simulink model "cPegasusAutopilot"  (R2020a)
settings: Solver=ode4  StartTime=0.0  StopTime=inf  FixedStep=0.01  RelTol=1e-3  EnableMultiTasking=on
undefined symbols (not defined in the file or in its folder): f, Ue
libraries: xpcutilitieslib x4, instrumentlib x2, simulink x1
settings Model: PauseTimes=88  Creator=Marcelo Henrique  LastModifiedBy=adalb
settings DataIOCC: LimitDataPoints=on  SaveFormat=Array  ReturnWorkspaceOutputs=off
settings OptimizationCC: LifeSpan=inf
settings DebuggingCC: AlgebraicLoopMsg=none  UnderspecifiedInitializationDetection=Classic  MergeDetectMultiDrivingBlocksExec=none  StateNameClashWarn=warning  SFUnexpectedBacktrackingDiag=warning  SFNoUnconditionalDefaultTransitionDiag=warning  ArithmeticOperatorsInVariantConditions=warning
settings HardwareCC: ProdBitPerPointer=32  ProdBitPerSizeT=32  ProdBitPerPtrDiffT=32  ProdLargestAtomicFloat=None  ProdIntDivRoundTo=Undefined  ProdEndianess=Unspecified  ProdWordSize=32  ProdHWDeviceType=32-bit Generic
settings ModelReferenceCC: PropagateSignalLabelsOutOfModel=off
settings SFSimCC: SimUseLocalCustomCode=off  CustomCodeUndefinedFunction=UseInterfaceOnly
settings RTWCC: RTWUseLocalCustomCode=off
settings CodeAppCC: StateflowObjectComments=on
settings GRTTargetCC: TargetLangStandard=C89/C90 (ANSI)
settings ConfigComp: CovMetricSettings=dw  CovHtmlReporting=on  CovSaveCumulativeToWorkspaceVar=on  CovSaveSingleToWorkspaceVar=on  CovExternalEMLEnable=off

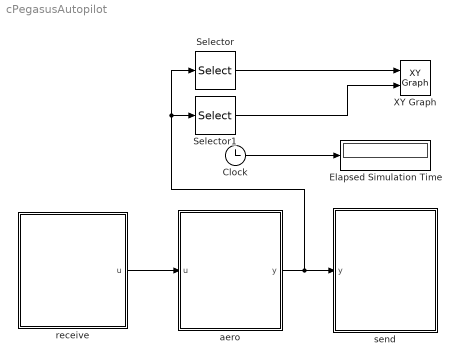
== system cPegasusAutopilot ==
  Clock : Clock
  Elapsed Simulation Time : Display
      settings: Decimation=2
  Selector : Selector  InputPortWidth=12  IndexOptions=Index vector (dialog)  Indices=[10]  OutputSizes=1
  Selector1 : Selector  InputPortWidth=12  IndexOptions=Index vector (dialog)  Indices=[11]  OutputSizes=1
  XY Graph : simulink/Sinks/XY Graph  xmin=-1500  xmax=1500  ymin=-1500  ymax=1500  st=-1
  aero : Subsystem
  receive : Subsystem
  send : Subsystem
  wires:
  aero/1(y) -> Selector1/1, Selector/1, send/1(y)
  receive/1(u) -> aero/1(u)
  Clock/1 -> Elapsed Simulation Time/1
  Selector/1 -> XY Graph/1
  Selector1/1 -> XY Graph/2

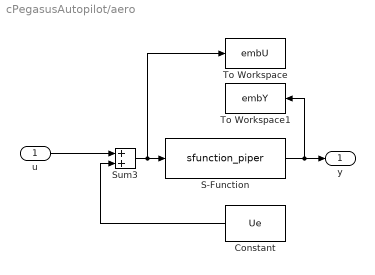
== system cPegasusAutopilot/aero ==
  u : Inport
  Constant : Constant  Value=Ue
  S-Function : S-Function  FunctionName=sfunction_piper  Parameters=par_gen,par_aero,par_prop, Xe  SFunctionDeploymentMode=off  EnableBusSupport=off
  Sum3 : Sum
  To Workspace : ToWorkspace  VariableName=embU  SaveFormat=Timeseries  SampleTime=-1
  To Workspace1 : ToWorkspace  VariableName=embY  SaveFormat=Timeseries  SampleTime=-1
  y : Outport
  wires:
  u/1 -> Sum3/1
  S-Function/1 -> To Workspace1/1, y/1
  Constant/1 -> Sum3/2
  Sum3/1 -> To Workspace/1, S-Function/1

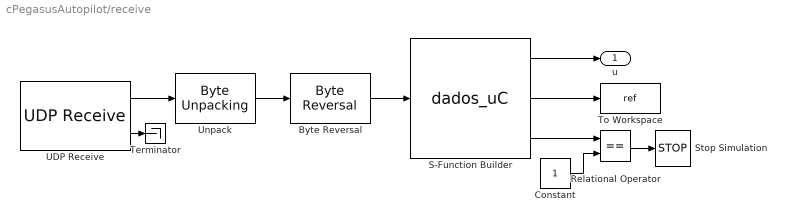
== system cPegasusAutopilot/receive ==
  Byte Reversal : xpcutilitieslib/Byte Reversal   numInp=1
      settings: SourceProductBaseCode=XP
  Constant : Constant
  Relational Operator : RelationalOperator  Operator===  OutDataTypeStr=boolean  RndMeth=Nearest
  S-Function Builder : S-Function  InitFcn=try, set_param(gcb,'FunctionName','dados_uC'), end  FunctionName=dados_uC  SFunctionModules=dados_uC_wrapper  SFunctionDeploymentMode=off  EnableBusSupport=off  mask(S-Function Builder){}
      mask help: Simulink:masks:SFunctionBuilder_MD
      mask init:
      | val = [[.9  0.75 0.75 1 1 .9 .9 1]',[1 1 0.75 0.75 .9 .9 1 .9]'];try , sys = get_param(gcb,'SfunBuilderFcnName');if isempty(sys), sys = get_param(gcb,'FunctionName'); end,catch, sys = get_param(gcb,'FunctionName'); end
      settings: CopyFcn=set_param(gcbh,'LinkStatus','none')  PreSaveFcn=try, set_param(gcb,'FunctionName','dados_uC'), end  OpenFcn=sfunctionwizard(gcbh)
      mask Display: plot(val(:,1),val(:,2)),disp(sys), port_label('input',1,'Pkt'), port_label('output',1,'u'), port_label('output',2,'WP'), port_label('output',3,'stop')
  Stop Simulation : Stop
  Terminator : Terminator
  To Workspace : ToWorkspace  VariableName=ref  SaveFormat=Timeseries  SampleTime=-1
  UDP Receive : instrumentlib/UDP Receive  Host=192.168.1.101  Port=45004  LocalPort=45000  EnablePortSharing=off  GetLatestData=off  DataSize=41  DataType=uint8  ASCIIFormatting=%f,  Terminator=LF  ByteOrder=BigEndian  EnableBlockingMode=off  Timeout=10  SampleTime=0.01  LocalAddress=0.0.0.0
  Unpack : xpcutilitieslib/Byte Unpacking   MaskUnpackedDataTypes={'uint8'}  MaskUnpackedDataSizes={[1 41]}  MaskAlignment=1
      settings: SourceProductBaseCode=XP
  u : Outport
  wires:
  UDP Receive/1 -> Unpack/1
  Unpack/1 -> Byte Reversal/1
  UDP Receive/2 -> Terminator/1
  S-Function Builder/1 -> u/1
  Relational Operator/1 -> Stop Simulation/1
  Constant/1 -> Relational Operator/2
  Byte Reversal/1 -> S-Function Builder/1
  S-Function Builder/3 -> Relational Operator/1
  S-Function Builder/2 -> To Workspace/1

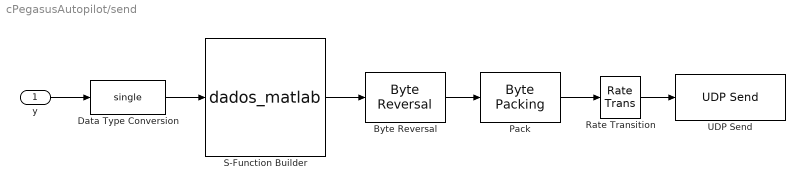
== system cPegasusAutopilot/send ==
  y : Inport
  Byte Reversal : xpcutilitieslib/Byte Reversal   numInp=1
      settings: SourceProductBaseCode=XP
  Data Type Conversion : DataTypeConversion  OutDataTypeStr=single
  Pack : xpcutilitieslib/Byte Packing   MaskPackedDataType=uint8  MaskUnpackedDataTypes={'uint8'}  MaskAlignment=1
  Rate Transition : RateTransition  OutPortSampleTime=0.01
  S-Function Builder : S-Function  InitFcn=try, set_param(gcb,'FunctionName','dados_matlab'), end  FunctionName=dados_matlab  SFunctionModules=dados_matlab_wrapper crc  SFunctionDeploymentMode=off  EnableBusSupport=off  mask(S-Function Builder){}
      mask help: Simulink:masks:SFunctionBuilder_MD
      mask init: same as cPegasusAutopilot/receive/S-Function Builder
      settings: CopyFcn=set_param(gcbh,'LinkStatus','none')  PreSaveFcn=try, set_param(gcb,'FunctionName','dados_matlab'), end  OpenFcn=sfunctionwizard(gcbh)
      mask Display: plot(val(:,1),val(:,2)),disp(sys), port_label('input',1,'y'), port_label('output',1,'Pkt')
  UDP Send : instrumentlib/UDP Send  Host=192.168.1.101  Port=45004  LocalPort=45001  EnablePortSharing=off  ByteOrder=BigEndian  OutputDatagramPacketSize=512  EnableBlockingMode=on  LocalAddress=0.0.0.0
  wires:
  Byte Reversal/1 -> Pack/1
  y/1 -> Data Type Conversion/1
  S-Function Builder/1 -> Byte Reversal/1
  Data Type Conversion/1 -> S-Function Builder/1
  Pack/1 -> Rate Transition/1
  Rate Transition/1 -> UDP Send/1
